simulink model "scoreV1"  (R2021a)
settings: Solver=VariableStepAuto  StartTime=0.0  StopTime=4000  MaxStep=10.0  RelTol=1e-3
model workspace (MAT data in the model file):
  Ts = 10
  amp = 1.1
  capacity = 100
  initial_available = 43
  limit = 200000
  lowSpaceRatio = 0.8
  moveQps = 0.052
  usedSize = 57
undefined symbols (not defined in the file or in its folder): DiscIntNeverNeededParam, hma_dens, hma_nums
libraries: pingcap x3
settings Model: Creator=tongjian  LastModifiedBy=tongjian

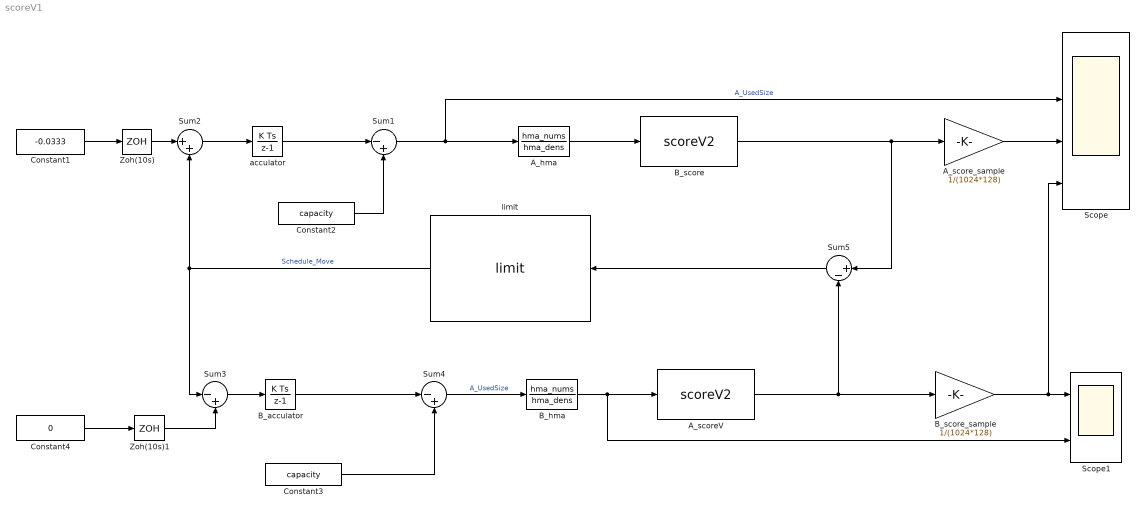
== system scoreV1 ==
  A_hma : DiscreteTransferFcn  Numerator=hma_nums  Denominator=hma_dens  InitialStates=initial_available  SampleTime=Ts
  A_scoreV : pingcap/scoreV2  g_lowSpaceRatio=lowSpaceRatio  g_amp=amp  g_capacity=capacity
  A_score_sample : Gain  Gain=1/(1024*128)
  B_acculator : DiscreteIntegrator  InitialCondition=initial_available  SampleTime=Ts  ICPrevOutput=DiscIntNeverNeededParam  ICPrevScaledInput=DiscIntNeverNeededParam
  B_hma : DiscreteTransferFcn  Numerator=hma_nums  Denominator=hma_dens  InitialStates=initial_available  SampleTime=Ts
  B_score : pingcap/scoreV2  g_lowSpaceRatio=lowSpaceRatio  g_amp=amp  g_capacity=capacity
  B_score_sample : Gain  Gain=1/(1024*128)
  Constant1 : Constant  Value=-0.0333
  Constant2 : Constant  Value=capacity
  Constant3 : Constant  Value=capacity
  Constant4 : Constant  Value=0
  Scope : Scope  NumInputPorts=4
  Scope1 : Scope  NumInputPorts=2
  Sum1 : Sum  Inputs=|-+
  Sum2 : Sum  Inputs=|++
  Sum3 : Sum  Inputs=|-+
  Sum4 : Sum  Inputs=|-+
  Sum5 : Sum  Inputs=|+-
  Zoh(10s) : ZeroOrderHold  Description=Zoh(10s)  SampleTime=10
  Zoh(10s)1 : ZeroOrderHold  Description=Zoh(10s)  SampleTime=10
  acculator : DiscreteIntegrator  InitialCondition=initial_available  SampleTime=Ts  ICPrevOutput=DiscIntNeverNeededParam  ICPrevScaledInput=DiscIntNeverNeededParam
  limit : pingcap/limit  g_limit=limit  g_value=moveQps
  wires:
  A_hma/1 -> B_score/1
  Sum2/1 -> acculator/1
  B_acculator/1 -> Sum4/1
  Zoh(10s)/1 -> Sum2/1
  acculator/1 -> Sum1/1
  Constant1/1 -> Zoh(10s)/1
  B_score_sample/1 -> Scope1/1, Scope/4
  Constant4/1 -> Zoh(10s)1/1
  Zoh(10s)1/1 -> Sum3/2
  A_scoreV/1 -> B_score_sample/1, Sum5/2
  B_score/1 -> A_score_sample/1, Sum5/1
  Constant3/1 -> Sum4/2
  B_hma/1 -> Scope1/2, A_scoreV/1
  Sum5/1 -> limit/1
  Sum4/1 -> B_hma/1  "A_UsedSize"
  A_score_sample/1 -> Scope/3
  Sum1/1 -> Scope/2, A_hma/1  "A_UsedSize"
  Constant2/1 -> Sum1/2
  Sum3/1 -> B_acculator/1
  limit/1 -> Sum2/2, Sum3/1  "Schedule_Move"
